simulink model "visismodelsubsystem"  (Simulink 6.4)
settings: Solver=FixedStepDiscrete  StartTime=0.0  StopTime=1039  FixedStep=sampleTime  RelTol=1e-3
libraries: vrlib x1
settings Model: LastModifiedBy=Roman

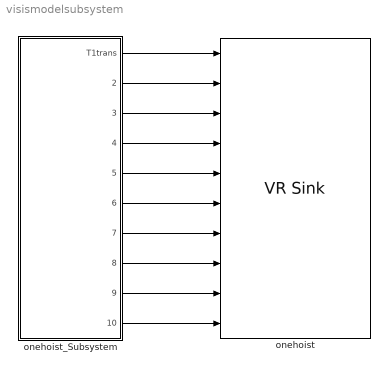
== system visismodelsubsystem ==
  onehoist_Subsystem : Subsystem
  onehoist : vrlib/VR Sink  SampleTime=1  ViewEnable=on  RemoteChange=off  RemoteView=on  FieldsWritten=T1.translation.3.1.double#T2.translation.3.1.double#T3.translation.3.1.double#T4.translation.3.1.double#Arm1.translation.3.1.double#Wrist1.translation.3.1.double#ArmStick1.height.1.1.double#Fingers1.translation.3.1.double#Upper_text.translation.3.1.double#Pointer.translation.3.1.double#  WorldFileName=onehoist.wrl  AutoView=on  FigureProperties={'Position', 'Record2DFileName'; [5,75,1270,350], '%f_anim_%n.avi'}
  wires:
  onehoist_Subsystem/1(Pointer) -> onehoist/1
  onehoist_Subsystem/2 -> onehoist/2
  onehoist_Subsystem/3 -> onehoist/3
  onehoist_Subsystem/4 -> onehoist/4
  onehoist_Subsystem/5 -> onehoist/5
  onehoist_Subsystem/6 -> onehoist/6
  onehoist_Subsystem/7 -> onehoist/7
  onehoist_Subsystem/8 -> onehoist/8
  onehoist_Subsystem/9 -> onehoist/9
  onehoist_Subsystem/10 -> onehoist/10

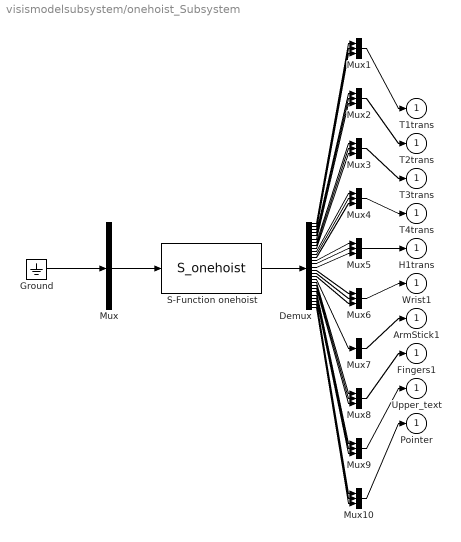
== system visismodelsubsystem/onehoist_Subsystem ==
  Demux : Demux  Outputs=28
  Mux : Mux  Inputs=1
  S-Function onehoist : S-Function  FunctionName=S_onehoist  Parameters=file(1:end-4),sampleTime,TS,period
  Ground : Ground
  T1trans : Outport
      settings: BusOutputAsStruct=off
  Mux{1..6,8..10} (9 alike) : Mux  Inputs=3
  T2trans : Outport
      settings: BusOutputAsStruct=off
  T3trans : Outport
      settings: BusOutputAsStruct=off
  T4trans : Outport
      settings: BusOutputAsStruct=off
  H1trans : Outport
      settings: BusOutputAsStruct=off
  Wrist1 : Outport
      settings: BusOutputAsStruct=off
  ArmStick1 : Outport
      settings: BusOutputAsStruct=off
  Mux7 : Mux  Inputs=1
  Fingers1 : Outport
      settings: BusOutputAsStruct=off
  Upper_text : Outport
      settings: BusOutputAsStruct=off
  Pointer : Outport
      settings: BusOutputAsStruct=off
  wires:
  Mux/1 -> S-Function onehoist/1
  S-Function onehoist/1 -> Demux/1
  Ground/1 -> Mux/1
  Mux1/1 -> T1trans/1
  Demux/1 -> Mux1/1
  Demux/2 -> Mux1/2
  Demux/3 -> Mux1/3
  Mux2/1 -> T2trans/1
  Demux/4 -> Mux2/1
  Demux/5 -> Mux2/2
  Demux/6 -> Mux2/3
  Mux3/1 -> T3trans/1
  Demux/7 -> Mux3/1
  Demux/8 -> Mux3/2
  Demux/9 -> Mux3/3
  Mux4/1 -> T4trans/1
  Demux/10 -> Mux4/1
  Demux/11 -> Mux4/2
  Demux/12 -> Mux4/3
  Mux5/1 -> H1trans/1
  Demux/13 -> Mux5/1
  Demux/14 -> Mux5/2
  Demux/15 -> Mux5/3
  Mux6/1 -> Wrist1/1
  Demux/16 -> Mux6/1
  Demux/17 -> Mux6/2
  Demux/18 -> Mux6/3
  Mux7/1 -> ArmStick1/1
  Demux/19 -> Mux7/1
  Mux8/1 -> Fingers1/1
  Demux/20 -> Mux8/1
  Demux/21 -> Mux8/2
  Demux/22 -> Mux8/3
  Mux9/1 -> Upper_text/1
  Demux/23 -> Mux9/1
  Demux/24 -> Mux9/2
  Demux/25 -> Mux9/3
  Mux10/1 -> Pointer/1
  Demux/26 -> Mux10/1
  Demux/27 -> Mux10/2
  Demux/28 -> Mux10/3
